simulink model "NCSEx1_sim"  (R2024b)
settings: Solver=VariableStepAuto  StartTime=0.0  StopTime=NCS.simTime  FixedStep=Td  RelTol=1e-3
InitFcn:
  | set_param(gcs, 'SimulationCommand', 'update')
values from neighbouring files (symbols this model uses):
  NCS = NcsStructureEx1(ncsPlant, 'simTime', simTime,                     'networkEffectsData', networkEffectsData,                     'controlParams', controlParams,                     'observerParams', observerParams)    [mainEx1.m]
undefined symbols (not defined in the file or in its folder): sfunchk
libraries: cstblocks x1, truetime x1
settings Model: Creator=jakob_ludwiger  LastModifiedBy=kala
settings SolverCC: AlgebraicLoopSolver=TrustRegion
settings DataIOCC: ReturnWorkspaceOutputs=off
settings DebuggingCC: UnconnectedInputMsg=warning  UnconnectedOutputMsg=warning  UnconnectedLineMsg=warning  ArithmeticOperatorsInVariantConditions=warning
settings ModelReferenceCC: EnableRefExpFcnMdlSchedulingChecks=on
settings SFSimCC: SimUseLocalCustomCode=off  CustomCodeUndefinedFunction=UseInterfaceOnly
settings RTWCC: RTWUseLocalCustomCode=off  GPUComputeCapability=3.5  DLArmComputeVersion=19.05
settings CodeAppCC: StateflowObjectComments=on

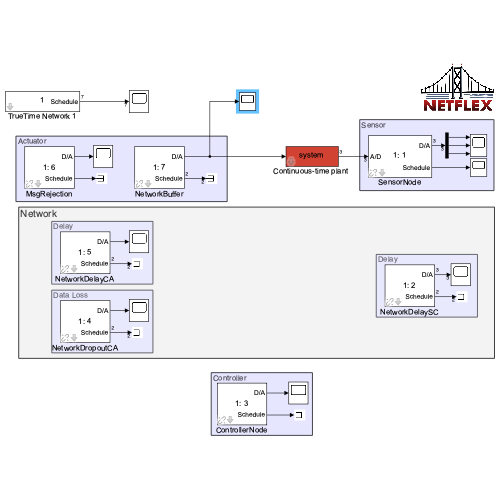
[thumbnail: Simulink's stored preview of the top-level diagram]
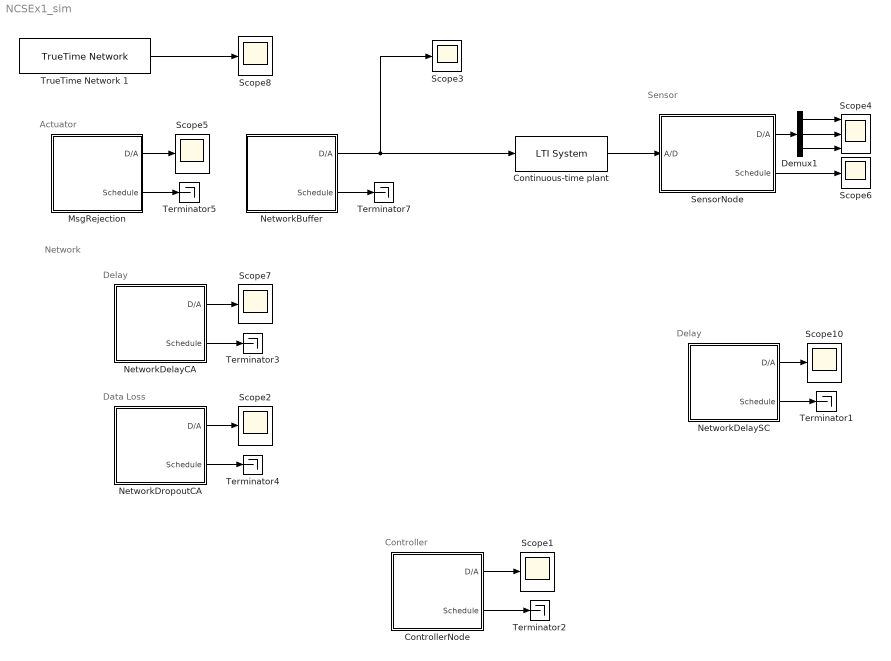
== system NCSEx1_sim ==
  note: Network
  note: Sensor
  note: Delay
  note: Delay
  note: Data Loss
  note: Actuator
  note: Controller
  "Continuous-time plant " : cstblocks/LTI System  sys=system  IC=initialState  PadeOrder=0
  ControllerNode : Subsystem  AncestorBlock=truetime/TrueTime Kernel  InitFcn=sfunchk(get_param(gcb,'sfun'));  mask{nodeObj=NCS.nodeMap('ControllerNode'), sfun=initFctWrapper, ntriggers=0, trigtype=falling, clockoffsetdrift=[0 0], schedoutput=on, battery=off, poweroutput=off, label=1: 3}
      mask prompts: nodeObj "Node Object"; sfun "Name of init function (MEX or MATLAB):"; ntriggers "Number of external triggers:"; trigtype "Trigger type:"; clockoffsetdrift "Local clock offset and drift:"; schedoutput "Show Schedule output port"; battery "Show Energy supply input port"; poweroutput "Show Power consumption output port"
      mask init:
      | set_param(gcb,'sfun', nodeObj.initFunctionWrapper)
      | %set_param(gcb,'args', [3 2])
      | args = nodeObj;
      | ninputsoutputs = [nodeObj.nIn nodeObj.nOut];
      | nwnodenbr = nodeObj.nodeNr;
      | ttkernel_callback(gcb,{sfun,args,ninputsoutputs,ntriggers,trigtype,nwnodenbr,clockoffsetdrift,schedoutput,battery,poweroutput})
      settings: ErrorFcn=ttkernel_error
      mask TypeOptions trigtype: rising | falling | either
      mask Display: disp(get_param(gcb,'label'))
  Demux1 : Demux  Outputs=3
  MsgRejection : Subsystem  AncestorBlock=truetime/TrueTime Kernel  InitFcn=sfunchk(get_param(gcb,'sfun'));  mask{nodeObj=NCS.nodeMap('MsgRejection'), sfun=initFctWrapper, ntriggers=0, trigtype=falling, clockoffsetdrift=[0 0], schedoutput=on, battery=off, poweroutput=off, label=1: 6}
      mask prompts: nodeObj "Node Object"; sfun "Name of init function (MEX or MATLAB):"; ntriggers "Number of external triggers:"; trigtype "Trigger type:"; clockoffsetdrift "Local clock offset and drift:"; schedoutput "Show Schedule output port"; battery "Show Energy supply input port"; poweroutput "Show Power consumption output port"
      mask init: same as NCSEx1_sim/ControllerNode
      settings: ErrorFcn=ttkernel_error
      mask TypeOptions trigtype: rising | falling | either
      mask Display: disp(get_param(gcb,'label'))
  NetworkBuffer : Subsystem  AncestorBlock=truetime/TrueTime Kernel  InitFcn=sfunchk(get_param(gcb,'sfun'));  mask{nodeObj=NCS.nodeMap('NetworkBuffer'), sfun=initFctWrapper, ntriggers=0, trigtype=falling, clockoffsetdrift=[0 0], schedoutput=on, battery=off, poweroutput=off, label=1: 7}
      mask prompts: nodeObj "Node Object"; sfun "Name of init function (MEX or MATLAB):"; ntriggers "Number of external triggers:"; trigtype "Trigger type:"; clockoffsetdrift "Local clock offset and drift:"; schedoutput "Show Schedule output port"; battery "Show Energy supply input port"; poweroutput "Show Power consumption output port"
      mask init: same as NCSEx1_sim/ControllerNode
      settings: ErrorFcn=ttkernel_error
      mask TypeOptions trigtype: rising | falling | either
      mask Display: disp(get_param(gcb,'label'))
  NetworkDelayCA : Subsystem  AncestorBlock=truetime/TrueTime Kernel  InitFcn=sfunchk(get_param(gcb,'sfun'));  mask{nodeObj=NCS.nodeMap('NetworkDelayCA'), sfun=initFctWrapper, ntriggers=0, trigtype=falling, clockoffsetdrift=[0 0], schedoutput=on, battery=off, poweroutput=off, label=1: 5}
      mask prompts: nodeObj "Node Object"; sfun "Name of init function (MEX or MATLAB):"; ntriggers "Number of external triggers:"; trigtype "Trigger type:"; clockoffsetdrift "Local clock offset and drift:"; schedoutput "Show Schedule output port"; battery "Show Energy supply input port"; poweroutput "Show Power consumption output port"
      mask init: same as NCSEx1_sim/ControllerNode
      settings: ErrorFcn=ttkernel_error
      mask TypeOptions trigtype: rising | falling | either
      mask Display: disp(get_param(gcb,'label'))
  NetworkDelaySC : Subsystem  AncestorBlock=truetime/TrueTime Kernel  InitFcn=sfunchk(get_param(gcb,'sfun'));  mask{nodeObj=NCS.nodeMap('NetworkDelaySC'), sfun=initFctWrapper, ntriggers=0, trigtype=falling, clockoffsetdrift=[0 0], schedoutput=on, battery=off, poweroutput=off, label=1: 2}
      mask prompts: nodeObj "Node Object"; sfun "Name of init function (MEX or MATLAB):"; ntriggers "Number of external triggers:"; trigtype "Trigger type:"; clockoffsetdrift "Local clock offset and drift:"; schedoutput "Show Schedule output port"; battery "Show Energy supply input port"; poweroutput "Show Power consumption output port"
      mask init: same as NCSEx1_sim/ControllerNode
      settings: ErrorFcn=ttkernel_error
      mask TypeOptions trigtype: rising | falling | either
      mask Display: disp(get_param(gcb,'label'))
  NetworkDropoutCA : Subsystem  AncestorBlock=truetime/TrueTime Kernel  InitFcn=sfunchk(get_param(gcb,'sfun'));  mask{nodeObj=NCS.nodeMap('NetworkDropoutCA'), sfun=initFctWrapper, ntriggers=0, trigtype=falling, clockoffsetdrift=[0 0], schedoutput=on, battery=off, poweroutput=off, label=1: 4}
      mask prompts: nodeObj "Node Object"; sfun "Name of init function (MEX or MATLAB):"; ntriggers "Number of external triggers:"; trigtype "Trigger type:"; clockoffsetdrift "Local clock offset and drift:"; schedoutput "Show Schedule output port"; battery "Show Energy supply input port"; poweroutput "Show Power consumption output port"
      mask init: same as NCSEx1_sim/ControllerNode
      settings: ErrorFcn=ttkernel_error
      mask TypeOptions trigtype: rising | falling | either
      mask Display: disp(get_param(gcb,'label'))
  Scope{1..3,5..8,10} (8 alike) : Scope
  Scope4 : Scope  NumInputPorts=3
  SensorNode : Subsystem  AncestorBlock=truetime/TrueTime Kernel  InitFcn=sfunchk(get_param(gcb,'sfun'));  mask{nodeObj=NCS.nodeMap('SensorNode'), sfun=initFctWrapper, ntriggers=0, trigtype=falling, clockoffsetdrift=[0 0], schedoutput=on, battery=off, poweroutput=off, label=1: 1}
      mask prompts: nodeObj "Node Object"; sfun "Name of init function (MEX or MATLAB):"; ntriggers "Number of external triggers:"; trigtype "Trigger type:"; clockoffsetdrift "Local clock offset and drift:"; schedoutput "Show Schedule output port"; battery "Show Energy supply input port"; poweroutput "Show Power consumption output port"
      mask init: same as NCSEx1_sim/ControllerNode
      settings: ErrorFcn=ttkernel_error
      mask TypeOptions trigtype: rising | falling | either
      mask Display: disp(get_param(gcb,'label'))
  Terminator{1..5,7} (6 alike) : Terminator
  TrueTime Network 1 : truetime/TrueTime Network  nwtype=CSMA/CD (Ethernet)  nwnbr=1  nnodes=NCS.getMaxNodeNr  rate=1e8  minsize=200  lossprob=0  seed=0  bandwidths=[0.5 0.5]  slotsize=512  schedule=[1 1 2]  memsize=80000  buftype=Common buffer  overflow=Retransmit  dynSchedule=0  miniSlotSize=0  NIT=0  QSortMode=FIFO  sync=0  irtSchedule=0  nrtLength=0  nodeGraph=0  scheduleoutput=on
  wires:
  SensorNode/2(Schedule) -> Scope6/1
  SensorNode/1(D/A) -> Demux1/1
  Demux1/1 -> Scope4/1
  Demux1/2 -> Scope4/2
  "Continuous-time plant "/1 -> SensorNode/1(A/D)
  NetworkBuffer/1(D/A) -> Scope3/1, "Continuous-time plant "/1
  TrueTime Network 1/1 -> Scope8/1
  NetworkDelaySC/2(Schedule) -> Terminator1/1
  NetworkDelaySC/1(D/A) -> Scope10/1
  NetworkDropoutCA/2(Schedule) -> Terminator4/1
  NetworkDropoutCA/1(D/A) -> Scope2/1
  NetworkDelayCA/1(D/A) -> Scope7/1
  NetworkDelayCA/2(Schedule) -> Terminator3/1
  MsgRejection/2(Schedule) -> Terminator5/1
  MsgRejection/1(D/A) -> Scope5/1
  NetworkBuffer/2(Schedule) -> Terminator7/1
  ControllerNode/1(D/A) -> Scope1/1
  ControllerNode/2(Schedule) -> Terminator2/1
  Demux1/3 -> Scope4/3

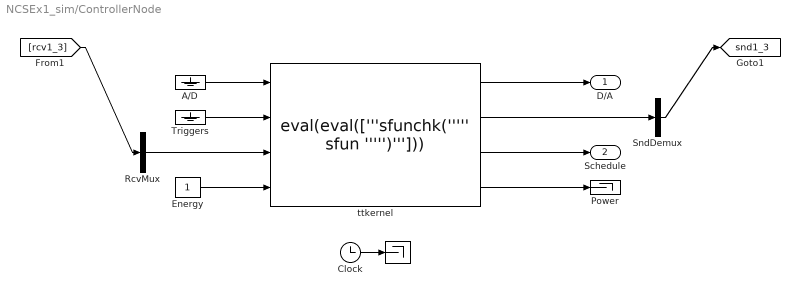
== system NCSEx1_sim/ControllerNode ==
  " " : Terminator
  A/D : Ground
  Clock : Clock
  Energy : Constant
  Power : Terminator
  RcvMux : Mux  Inputs=1
  SndDemux : Demux  Outputs=1
      settings: DisplayOption=none
  Triggers : Ground
  ttkernel : S-Function  FunctionName=eval(eval(['''sfunchk(''''' sfun ''''')''']))  Parameters=sfun, args, ninputsoutputs, ntriggers, trigtype, nwnodenbr, clockoffsetdrift  SFunctionDeploymentMode=off  EnableBusSupport=off
  D/A : Outport
  Schedule : Outport  Port=2
  tag scope: snd1_3=global
  wires:
  ttkernel/4 -> Power/1
  Energy/1 -> ttkernel/4
  A/D/1 -> ttkernel/1
  ttkernel/2 -> SndDemux/1
  ttkernel/1 -> D/A/1
  ttkernel/3 -> Schedule/1
  Triggers/1 -> ttkernel/2
  RcvMux/1 -> ttkernel/3
  Clock/1 -> " "/1
  [rcv1_3] -> RcvMux/1
  SndDemux/1 -> [snd1_3]

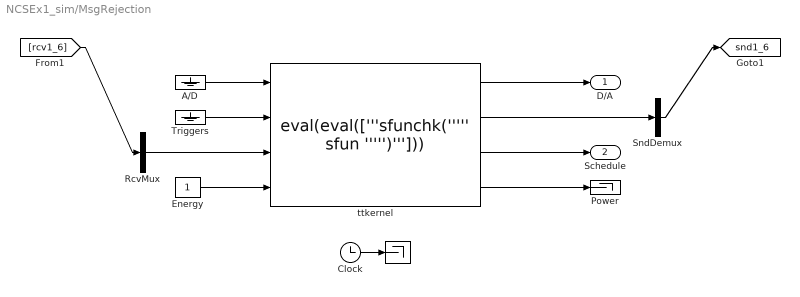
== system NCSEx1_sim/MsgRejection ==
  " " : Terminator
  A/D : Ground
  Clock : Clock
  Energy : Constant
  Power : Terminator
  RcvMux : Mux  Inputs=1
  SndDemux : Demux  Outputs=1
      settings: DisplayOption=none
  Triggers : Ground
  ttkernel : S-Function  FunctionName=eval(eval(['''sfunchk(''''' sfun ''''')''']))  Parameters=sfun, args, ninputsoutputs, ntriggers, trigtype, nwnodenbr, clockoffsetdrift  SFunctionDeploymentMode=off  EnableBusSupport=off
  D/A : Outport
  Schedule : Outport  Port=2
  tag scope: snd1_6=global
  wires:
  Clock/1 -> " "/1
  RcvMux/1 -> ttkernel/3
  Triggers/1 -> ttkernel/2
  ttkernel/3 -> Schedule/1
  ttkernel/1 -> D/A/1
  ttkernel/2 -> SndDemux/1
  A/D/1 -> ttkernel/1
  Energy/1 -> ttkernel/4
  ttkernel/4 -> Power/1
  [rcv1_6] -> RcvMux/1
  SndDemux/1 -> [snd1_6]

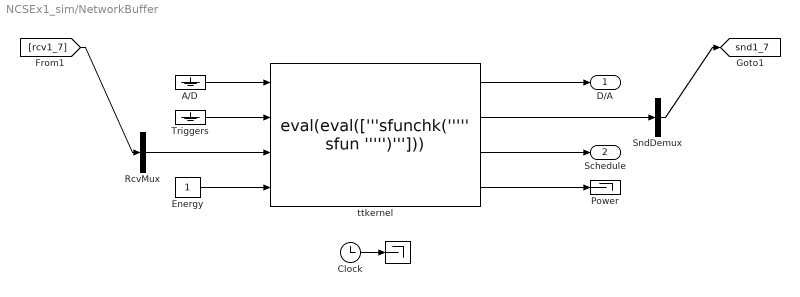
== system NCSEx1_sim/NetworkBuffer ==
  " " : Terminator
  A/D : Ground
  Clock : Clock
  Energy : Constant
  Power : Terminator
  RcvMux : Mux  Inputs=1
  SndDemux : Demux  Outputs=1
      settings: DisplayOption=none
  Triggers : Ground
  ttkernel : S-Function  FunctionName=eval(eval(['''sfunchk(''''' sfun ''''')''']))  Parameters=sfun, args, ninputsoutputs, ntriggers, trigtype, nwnodenbr, clockoffsetdrift  SFunctionDeploymentMode=off  EnableBusSupport=off
  D/A : Outport
  Schedule : Outport  Port=2
  tag scope: snd1_7=global
  wires:
  ttkernel/4 -> Power/1
  Energy/1 -> ttkernel/4
  A/D/1 -> ttkernel/1
  ttkernel/2 -> SndDemux/1
  ttkernel/1 -> D/A/1
  ttkernel/3 -> Schedule/1
  Triggers/1 -> ttkernel/2
  RcvMux/1 -> ttkernel/3
  Clock/1 -> " "/1
  [rcv1_7] -> RcvMux/1
  SndDemux/1 -> [snd1_7]

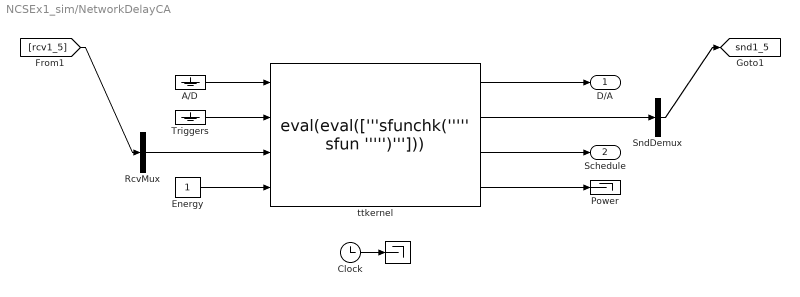
== system NCSEx1_sim/NetworkDelayCA ==
  " " : Terminator
  A/D : Ground
  Clock : Clock
  Energy : Constant
  Power : Terminator
  RcvMux : Mux  Inputs=1
  SndDemux : Demux  Outputs=1
      settings: DisplayOption=none
  Triggers : Ground
  ttkernel : S-Function  FunctionName=eval(eval(['''sfunchk(''''' sfun ''''')''']))  Parameters=sfun, args, ninputsoutputs, ntriggers, trigtype, nwnodenbr, clockoffsetdrift  SFunctionDeploymentMode=off  EnableBusSupport=off
  D/A : Outport
  Schedule : Outport  Port=2
  tag scope: snd1_5=global
  wires:
  ttkernel/4 -> Power/1
  Energy/1 -> ttkernel/4
  A/D/1 -> ttkernel/1
  ttkernel/2 -> SndDemux/1
  ttkernel/1 -> D/A/1
  ttkernel/3 -> Schedule/1
  Triggers/1 -> ttkernel/2
  RcvMux/1 -> ttkernel/3
  Clock/1 -> " "/1
  [rcv1_5] -> RcvMux/1
  SndDemux/1 -> [snd1_5]

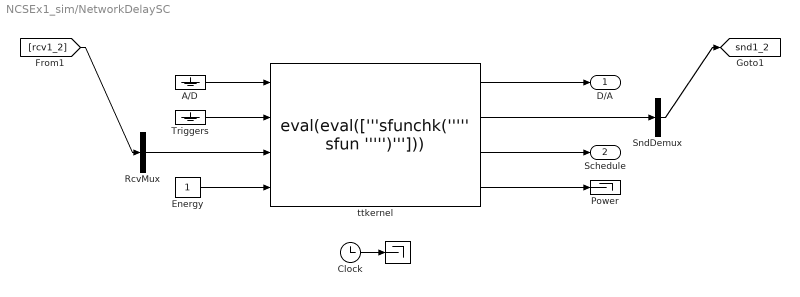
== system NCSEx1_sim/NetworkDelaySC ==
  " " : Terminator
  A/D : Ground
  Clock : Clock
  Energy : Constant
  Power : Terminator
  RcvMux : Mux  Inputs=1
  SndDemux : Demux  Outputs=1
      settings: DisplayOption=none
  Triggers : Ground
  ttkernel : S-Function  FunctionName=eval(eval(['''sfunchk(''''' sfun ''''')''']))  Parameters=sfun, args, ninputsoutputs, ntriggers, trigtype, nwnodenbr, clockoffsetdrift  SFunctionDeploymentMode=off  EnableBusSupport=off
  D/A : Outport
  Schedule : Outport  Port=2
  tag scope: snd1_2=global
  wires:
  Clock/1 -> " "/1
  RcvMux/1 -> ttkernel/3
  Triggers/1 -> ttkernel/2
  ttkernel/3 -> Schedule/1
  ttkernel/1 -> D/A/1
  ttkernel/2 -> SndDemux/1
  A/D/1 -> ttkernel/1
  Energy/1 -> ttkernel/4
  ttkernel/4 -> Power/1
  [rcv1_2] -> RcvMux/1
  SndDemux/1 -> [snd1_2]

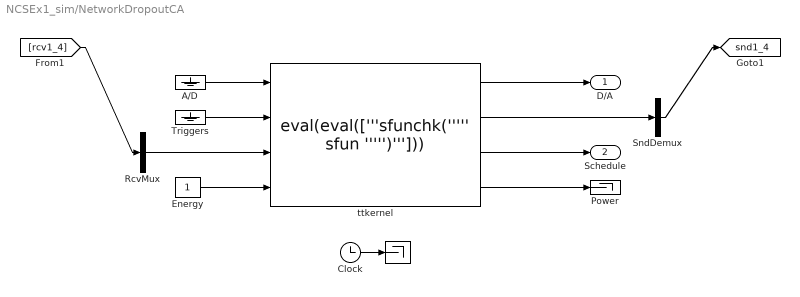
== system NCSEx1_sim/NetworkDropoutCA ==
  " " : Terminator
  A/D : Ground
  Clock : Clock
  Energy : Constant
  Power : Terminator
  RcvMux : Mux  Inputs=1
  SndDemux : Demux  Outputs=1
      settings: DisplayOption=none
  Triggers : Ground
  ttkernel : S-Function  FunctionName=eval(eval(['''sfunchk(''''' sfun ''''')''']))  Parameters=sfun, args, ninputsoutputs, ntriggers, trigtype, nwnodenbr, clockoffsetdrift  SFunctionDeploymentMode=off  EnableBusSupport=off
  D/A : Outport
  Schedule : Outport  Port=2
  tag scope: snd1_4=global
  wires:
  Clock/1 -> " "/1
  RcvMux/1 -> ttkernel/3
  Triggers/1 -> ttkernel/2
  ttkernel/3 -> Schedule/1
  ttkernel/1 -> D/A/1
  ttkernel/2 -> SndDemux/1
  A/D/1 -> ttkernel/1
  Energy/1 -> ttkernel/4
  ttkernel/4 -> Power/1
  [rcv1_4] -> RcvMux/1
  SndDemux/1 -> [snd1_4]

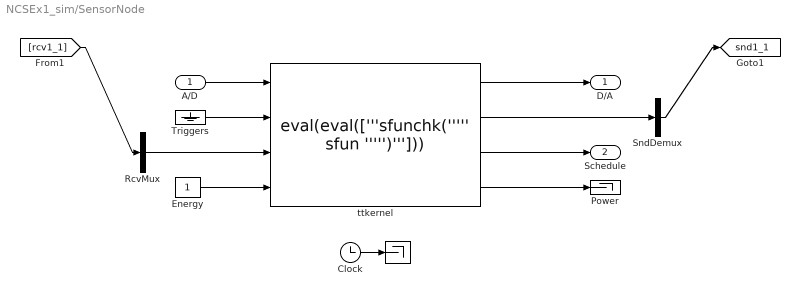
== system NCSEx1_sim/SensorNode ==
  A/D : Inport
  " " : Terminator
  Clock : Clock
  Energy : Constant
  Power : Terminator
  RcvMux : Mux  Inputs=1
  SndDemux : Demux  Outputs=1
      settings: DisplayOption=none
  Triggers : Ground
  ttkernel : S-Function  FunctionName=eval(eval(['''sfunchk(''''' sfun ''''')''']))  Parameters=sfun, args, ninputsoutputs, ntriggers, trigtype, nwnodenbr, clockoffsetdrift  SFunctionDeploymentMode=off  EnableBusSupport=off
  D/A : Outport
  Schedule : Outport  Port=2
  tag scope: snd1_1=global
  wires:
  ttkernel/4 -> Power/1
  Energy/1 -> ttkernel/4
  A/D/1 -> ttkernel/1
  ttkernel/2 -> SndDemux/1
  ttkernel/1 -> D/A/1
  ttkernel/3 -> Schedule/1
  Triggers/1 -> ttkernel/2
  RcvMux/1 -> ttkernel/3
  Clock/1 -> " "/1
  [rcv1_1] -> RcvMux/1
  SndDemux/1 -> [snd1_1]
